simulink model "parcial_SophiaUpegui"  (R2022b)
settings: Solver=VariableStepAuto  StartTime=0.0  StopTime=800  RelTol=1e-3
libraries: simulink x1
settings Model: Creator=Camila  LastModifiedBy=sophy
settings SolverCC: MaxZcPerStep=1
settings ModelReferenceCC: EnableRefExpFcnMdlSchedulingChecks=on

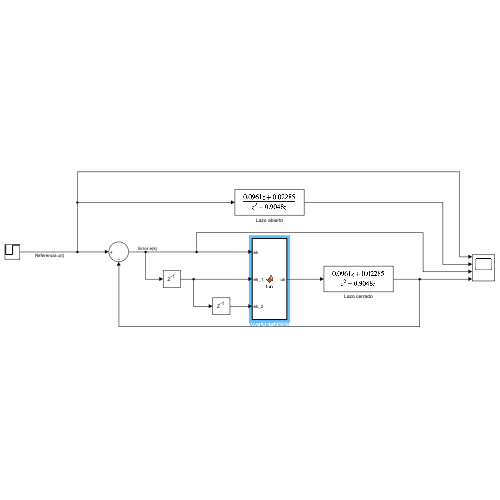
[thumbnail: Simulink's stored preview of the top-level diagram]
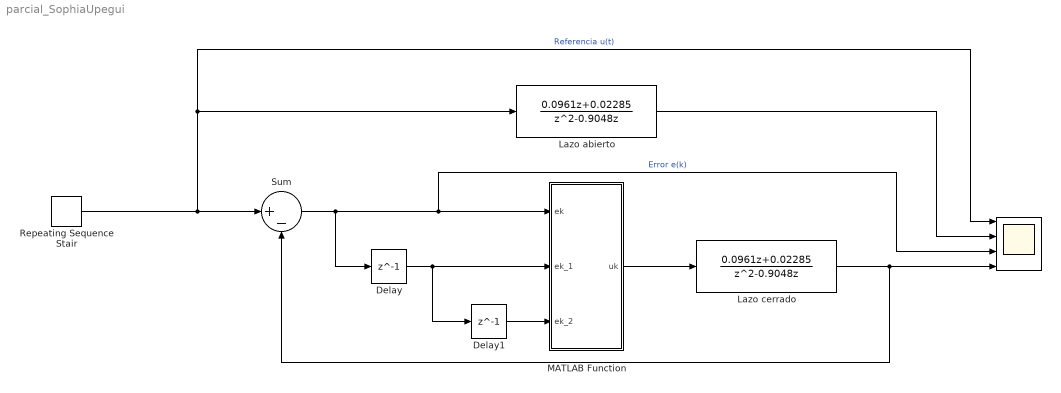
== system parcial_SophiaUpegui ==
  "  " : Scope  NumInputPorts=4
  Delay : Delay  DelayLength=1  InitialCondition=0  SampleTime=2.5
  Delay1 : Delay  DelayLength=1  InitialCondition=0  SampleTime=2.5
  Lazo abierto : DiscreteTransferFcn  Numerator=[0.0961 0.02285]  Denominator=[1 -0.9048 0]  SampleTime=2.5
  Lazo cerrado : DiscreteTransferFcn  Numerator=[0.0961 0.02285]  Denominator=[1 -0.9048 0]  SampleTime=2.5
  MATLAB Function : MATLAB Function  TreatAsAtomicUnit=on
  Repeating Sequence Stair : simulink/Sources/Repeating Sequence Stair  OutValues=[10 20].'  tsamp=400  OutMin=[]  OutMax=[]  OutDataTypeStr=double  OutputDataTypeScalingMode=double  OutDataType=fixdt(0,8)  ConRadixGroup=Best Precision: Vector-wise  OutScaling=2^-12
  Sum : Sum  Inputs=|+-
  wires:
  Lazo cerrado/1 -> Sum/2, "  "/4
  MATLAB Function/1(uk) -> Lazo cerrado/1
  Delay/1 -> Delay1/1, MATLAB Function/2(ek_1)
  Delay1/1 -> MATLAB Function/3(ek_2)
  Lazo abierto/1 -> "  "/2
  Repeating Sequence Stair/1 -> "  "/1, Lazo abierto/1, Sum/1  "Referencia u(t)"
  Sum/1 -> Delay/1, "  "/3, MATLAB Function/1(ek)  "Error e(k)"

== matlab function parcial_SophiaUpegui/MATLAB Function ==
  data: ek input; uk output; ek_1 input; ek_2 input
function uk = fcn(ek, ek_1, ek_2)

persistent cant_n1 cant_n2...
    W_c1 W_c2 W_c3...
    n e_c3 e_c2 e_c1 ...
    Yp1 Yt1 Yp2 Yt2 Yp3 Yt3 

if isempty(W_c1) 
    
    % Neuronas
    cant_n1 = 6; 
    cant_n2 = 3;
    
    % Factor de aprendizaje
    n= 0.076;

    % Pesos
    W_c1 = rand(cant_n1, 3); 
    W_c2 = rand(cant_n2,cant_n1);
    W_c3 = rand(1, cant_n2);
    
    % Salidas
    Yp1 = zeros(1,cant_n1); Yt1= zeros(1,cant_n1);
    Yp2 = zeros(1,cant_n2); Yt2= zeros(1,cant_n2);
    Yp3 = 0; 
    Yt3 = 0;
    
    %Error
    e_c3 = 0; 
    e_c2 = zeros(1,cant_n2); 
    e_c1 = zeros(1,cant_n1); 

end

% Normalizar
e = [ek; ek_1; ek_2];
e_max = max(e); 
e_min = min(e);

if e_max == e_min
   x = [ek, ek_1, ek_2]./e_max;
else
   x = (e - e_min) ./ (e_max - e_min);
end

% Recorrer capas
% Capa oculta 1
Yp1 = W_c1*x; 
Yt1 = sigmoide(Yp1); 

% Capa oculta 2
for i=1:cant_n2 
    Yp2 =(W_c2*Yt1');
    Yt2(i)= sigmoide(Yp2(i));
end
    
% Capa salida 
Yp3 = W_c3*Yt2'; 
Yt3 = sigmoide(Yp3)

% Error
e_c3 = ek;
e_c2 = e_c3*W_c3;
e_c1 = e_c2*W_c2;

% Actualizo pesos
for i = 1:cant_n1
    for j = 1:cant_n2
        d_sig1 = (exp(-Yt1(j)))/((1+exp(-Yt1(j)))^2);
        W_c1(i,j) = W_c1(i,j) + n*e_c1(i)*d_sig1*x(j); 
    end
end

for i = 1:cant_n2
    for j = 1:cant_n1
        d_sig2 = (exp(-Yt2(i)))/((1+exp(-Yt2(i)))^2);
        W_c2(i,j)= W_c2(i,j) + n*e_c2(i)*d_sig2*Yt1(j); 
    end
end  

for j = 1:cant_n2
    d_sig3 = (exp(-Yt3))/((1+exp(-Yt3))^2);
    W_c3(j) = W_c3(j) + n*e_c3*d_sig3*Yt2(j); 
end

% Actualizo taza de aprendizaje
n = n+(0.000009*ek);

% Salida
uk = Yt3*16

end

function yt = sigmoide(yp)
    yt = 1/(1+exp(-yp))
end
